simulink model "lab1simulink"  (R2022a)
settings: Solver=VariableStepAuto  StartTime=0.0  StopTime=10.0  RelTol=1e-3
settings Model: Creator=wusamson  LastModifiedBy=wusamson

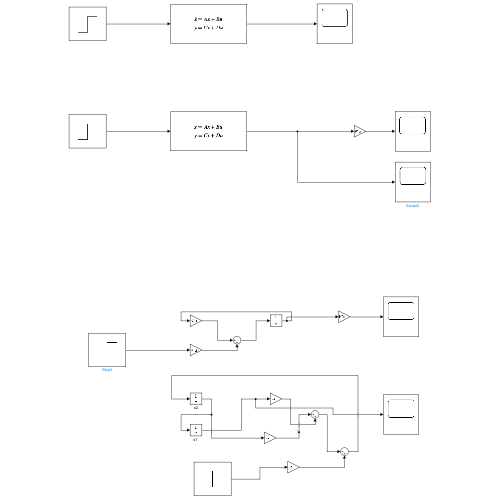
[thumbnail: Simulink's stored preview of the top-level diagram]
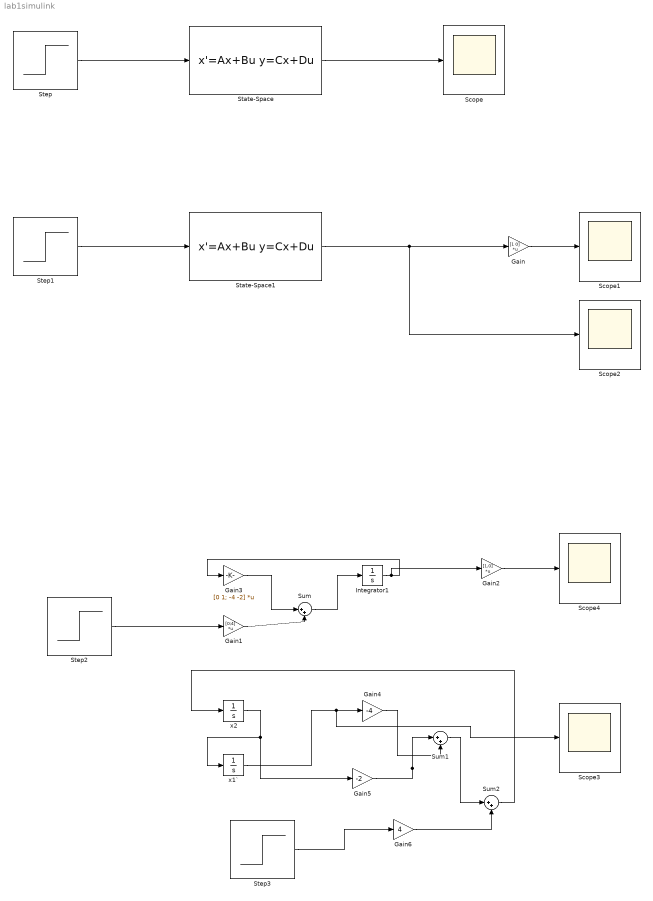
== system lab1simulink ==
  Gain : Gain  Gain=[1 0]  Multiplication=Matrix(K*u)
  Gain1 : Gain  Gain=[0;4]  Multiplication=Matrix(K*u)
  Gain2 : Gain  Gain=[1,0]  Multiplication=Matrix(K*u)
  Gain3 : Gain  Gain=[0 1; -4 -2]  Multiplication=Matrix(K*u)
  Gain4 : Gain  Gain=-4
  Gain5 : Gain  Gain=-2
  Gain6 : Gain  Gain=4
  Integrator1 : Integrator
  Scope{,1..4} (5 alike) : Scope
  State-Space : StateSpace  A=[0 1; -4 -2]  B=[0 ; 4]  C=[1 0]  D=[0]  InitialCondition=0
  State-Space1 : StateSpace  A=[0 1; -4 -2]  B=[0 ; 4]  C=[1 0; 0 1]  D=[0;0]  InitialCondition=0
  Step{,1..3} (4 alike) : Step  SampleTime=0
  Sum : Sum  Inputs=|++
  Sum1 : Sum  Inputs=|++
  Sum2 : Sum  Inputs=|++
  x1` : Integrator
  x2 : Integrator
  wires:
  Step/1 -> State-Space/1
  State-Space/1 -> Scope/1
  Step1/1 -> State-Space1/1
  State-Space1/1 -> Scope2/1, Gain/1
  Gain/1 -> Scope1/1
  Step2/1 -> Gain1/1
  Integrator1/1 -> Gain2/1, Gain3/1
  Gain1/1 -> Sum/2
  Gain3/1 -> Sum/1
  Sum/1 -> Integrator1/1
  Gain2/1 -> Scope4/1
  x2/1 -> Gain5/1, x1`/1
  x1`/1 -> Scope3/1, Gain4/1
  Gain5/1 -> Sum1/1
  Gain4/1 -> Sum1/2
  Sum1/1 -> Sum2/1
  Step3/1 -> Gain6/1
  Gain6/1 -> Sum2/2
  Sum2/1 -> x2/1
